simulink library "Heat"  (R2019a)
settings: Solver=VariableStepAuto  StartTime=0.0  StopTime=10.0  RelTol=1e-3
PreLoadFcn:
  | load HeatShield_Models_Greybox.mat
undefined symbols (not defined in the file or in its folder): model, Ta
libraries: arduinolib x2, $bdroot x2, slident x1
settings Model: Creator=Gergely  LastModifiedBy=Gergely
settings DataIOCC: ReturnWorkspaceOutputs=off
settings DebuggingCC: PregeneratedLibrarySubsystemCodeDiagnostic=none  ArithmeticOperatorsInVariantConditions=warning
settings SFSimCC: SimUseLocalCustomCode=off
settings RTWCC: RTWUseLocalCustomCode=off

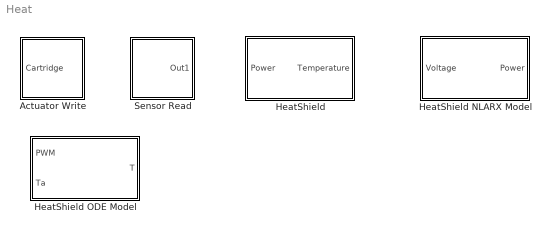
== system Heat ==
  Actuator Write : Subsystem
      mask DialogControl DescGroupVar Prompt: HeatShield Heating Cartridge
      mask DialogControl DescTextVar Prompt: Sets power to the heating cartridge in the heating block of the HeatShield. Expects input in the range of 0-100%.
      mask Display: image('assets\HeatShield_Cartridge.svg');
  HeatShield : Subsystem  mask{Ts=2.0}
      mask prompts: Ts "Sampling period (s):"
      mask DialogControl DescGroupVar Prompt: HeatShield
      mask DialogControl DescTextVar Prompt: The block represents the HeatShield device. It accepts an input signal for powering the heating cartridge in the range of 0-100% and outputs a sensor reading in degrees Celsius. The block requires a sampling period.
      mask Display: image('assets\HeatShield.svg');
  HeatShield NLARX Model : Subsystem
      mask init:
      | load HeatShield_Models_Blackbox.mat
      mask DialogControl DescGroupVar Prompt: HeatShield Nonlinear ARX model
      mask DialogControl DescTextVar Prompt: The block represents the HeatShield device. It accepts an input signal for powering the heating cartridge in the range of 0-100% and outputs a sensor reading in degrees Celsius.
      mask Display:
      | image('assets\HeatShield_NLARX.svg');
      | port_label('input', 1, 'u [%]');
      | port_label('output', 1,'T [C]');
  HeatShield ODE Model : Subsystem  mask{mc=model.Parameters(2).Value, hA=model.Parameters(1).Value, VR=model.Parameters(3).Value}
      mask prompts: mc "Heat capacity (m·c) [J/K]:"; hA "Convective resistance (h·A) [W·K]:"; VR "Joule heating (V²2/R) [V/Ω]:"
      mask init:
      | load HeatShield_Models_Greybox.mat;
      mask DialogControl DescGroupVar Prompt: HeatShield First Principles Model
      mask DialogControl DescTextVar Prompt: The block represents the HeatShield device. It accepts an input signal for powering the heating cartridge in the range of 0-100% and the ambient temperature, which may also change. It outputs a sensor reading in degrees Celsius.
      mask Display:
      | image('assets\HeatShield_ODE.svg');
      | port_label('input', 2, 'Ta [C]');
      | port_label('input', 1, 'u [%]');
      | port_label('output', 1,'T [C]');
  Sensor Read : Subsystem  mask{ReadoutRadio=Temperature, R0=100000, beta=3950, T0=25.0, Vin=5.0, R1=100000, Ts=2}
      mask prompts: ReadoutRadio "Readout type"; R0 "Nominal Resistance (Ω):"; beta "Beta constant:"; T0 "Reference temperature: (°C)"; Vin "Reference voltage (V):"; R1 "Reference resistance (Ω):"; Ts "Sample time (s):"
      mask init:
      | ADC_Gain=(5.0/1024);
      mask TypeOptions ReadoutRadio: Temperature | Resistance | Voltage | ADC levels
      mask DialogControl DescGroupVar Prompt: HeatShield Thermistor
      mask DialogControl DescTextVar Prompt: The block represents the main thermistor in the heating block of the HeatShield device. You may select the type of output, depending on your needs. The pre-filled parameters for the thermistor and the connected voltage divider should not be modified.
      mask DialogControl Container2 Prompt: Thermistor
      mask DialogControl Container5 Prompt: Voltage divider
      mask DialogControl Container3 Prompt: Parameters
      mask Display: image('assets\HeatShield_Thermistor.svg');

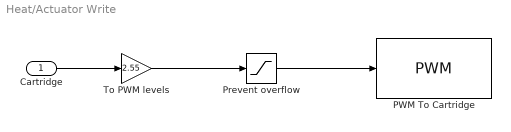
== system Heat/Actuator Write ==
  Cartridge : Inport
  PWM To Cartridge : arduinolib/PWM  pinNumber=3  EnableInputFrequency=off  InitialFrequency=2000  InitialDutyCycle=0  NotificationType=None  blockPlatform=arduino
  Prevent overflow : Saturate  UpperLimit=255  LowerLimit=0
  To PWM levels : Gain  Gain=2.55
  wires:
  To PWM levels/1 -> Prevent overflow/1
  Prevent overflow/1 -> PWM To Cartridge/1
  Cartridge/1 -> To PWM levels/1

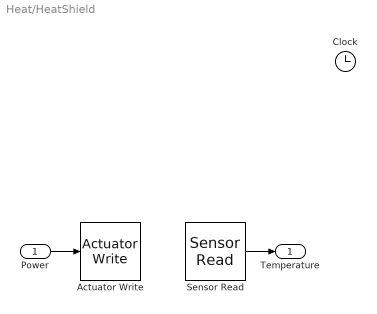
== system Heat/HeatShield ==
  Power : Inport
  Actuator Write : $bdroot/Actuator Write
  Clock : Clock
  Sensor Read : $bdroot/Sensor Read  ReadoutRadio=Temperature  R0=100000  beta=3950  T0=25.0  Vin=5.0  R1=100000  Ts=2
  Temperature : Outport
  wires:
  Sensor Read/1 -> Temperature/1
  Power/1 -> Actuator Write/1

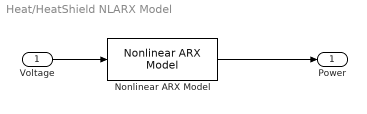
== system Heat/HeatShield NLARX Model ==
  Voltage : Inport
  Nonlinear ARX Model : slident/Models/Nonlinear ARX Model  sys=model_nlarx  ICspec=Input and output values  X0=0  U0=25  Y0=31
      settings: SourceProductName=System Identification Toolbox  SourceProductBaseCode=ID
  Power : Outport
  wires:
  Nonlinear ARX Model/1 -> Power/1
  Voltage/1 -> Nonlinear ARX Model/1

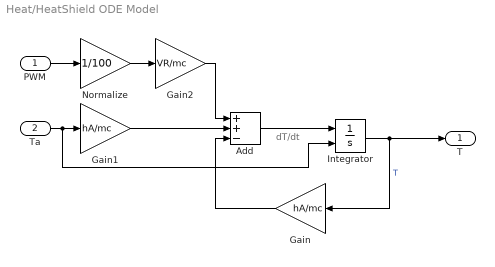
== system Heat/HeatShield ODE Model ==
  note: dT/dt
  PWM : Inport
  Ta : Inport  Port=2
  Add : Sum  Inputs=++-
  Gain : Gain  Gain=hA/mc
  Gain1 : Gain  Gain=hA/mc
  Gain2 : Gain  Gain=VR/mc
  Integrator : Integrator  InitialConditionSource=external  InitialCondition=Ta
  Normalize : Gain  Gain=1/100
  T : Outport
  wires:
  Integrator/1 -> T/1, Gain/1  "T"
  PWM/1 -> Normalize/1
  Ta/1 -> Integrator/2, Gain1/1
  Gain1/1 -> Add/2
  Add/1 -> Integrator/1
  Normalize/1 -> Gain2/1
  Gain2/1 -> Add/1
  Gain/1 -> Add/3

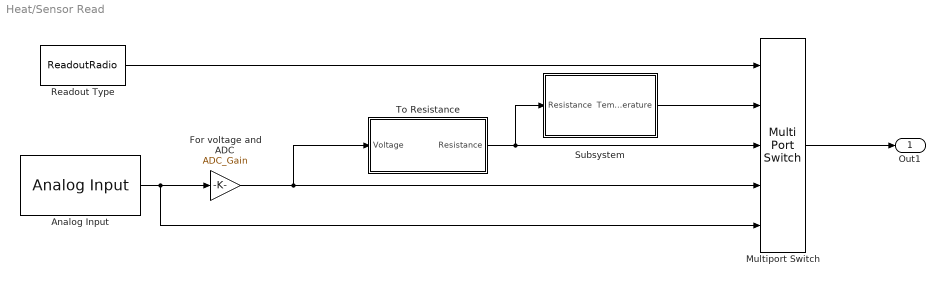
== system Heat/Sensor Read ==
  Analog Input : arduinolib/Analog Input  pinNumber=0  ReadResultsOnly=off  ConversionTriggerSource=Software  ExternalTriggerType=uint32(0)  OutputDataType=uint16  EnableConversionCompleteNotify=off  EnableOuputStatus=off  SampleTime=Ts  blockPlatform=arduino
  For voltage and ADC : Gain  Gain=ADC_Gain
  Multiport Switch : MultiPortSwitch  Inputs=4
  Readout Type : Constant  Value=ReadoutRadio  SampleTime=Ts
  Subsystem : Subsystem
  To Resistance : Subsystem
  Out1 : Outport
  wires:
  For voltage and ADC/1 -> To Resistance/1(Voltage), Multiport Switch/4
  Analog Input/1 -> Multiport Switch/5, For voltage and ADC/1
  Readout Type/1 -> Multiport Switch/1
  Multiport Switch/1 -> Out1/1
  To Resistance/1(Resistance) -> Subsystem/1(Resistance), Multiport Switch/3
  Subsystem/1(Temperature) -> Multiport Switch/2

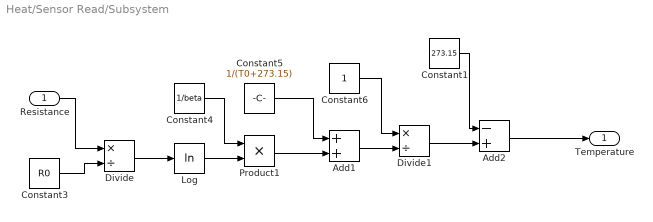
== system Heat/Sensor Read/Subsystem ==
  Resistance : Inport
  Add1 : Sum
  Add2 : Sum  Inputs=-+
  Constant1 : Constant  Value=273.15  SampleTime=Ts
  Constant3 : Constant  Value=R0  SampleTime=Ts
  Constant4 : Constant  Value=1/beta  SampleTime=Ts
  Constant5 : Constant  Value=1/(T0+273.15)  SampleTime=Ts
  Constant6 : Constant  SampleTime=Ts
  Divide : Product  Inputs=*/
  Divide1 : Product  Inputs=*/
  Log : Math  Operator=log  SaturateOnIntegerOverflow=on
  Product1 : Product
  Temperature : Outport
  wires:
  Log/1 -> Product1/2
  Constant3/1 -> Divide/2
  Constant6/1 -> Divide1/1
  Divide1/1 -> Add2/2
  Constant1/1 -> Add2/1
  Add1/1 -> Divide1/2
  Product1/1 -> Add1/2
  Constant4/1 -> Product1/1
  Divide/1 -> Log/1
  Constant5/1 -> Add1/1
  Add2/1 -> Temperature/1
  Resistance/1 -> Divide/1

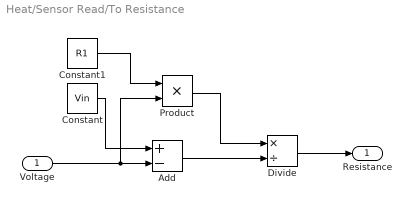
== system Heat/Sensor Read/To Resistance ==
  Voltage : Inport
  Add : Sum  Inputs=+-
  Constant : Constant  Value=Vin  SampleTime=Ts
  Constant1 : Constant  Value=R1  SampleTime=Ts
  Divide : Product  Inputs=*/
  Product : Product
  Resistance : Outport
  wires:
  Constant1/1 -> Product/1
  Constant/1 -> Add/1
  Voltage/1 -> Product/2, Add/2
  Divide/1 -> Resistance/1
  Add/1 -> Divide/2
  Product/1 -> Divide/1
